simulink model "P2lab"  (Simulink 10.3)
settings: Solver=VariableStepAuto  StartTime=0.0  StopTime=Tfin  FixedStep=dt  MaxStep=dtmax  RelTol=1e-3  EnableMultiTasking=on
values from neighbouring files (symbols this model uses):
  a = 1    [P2_1b.m]    (also in P2_laboratorio.m)
  A0 = 1    [P2_1b.m]    (also in P2_laboratorio.m)
  b = 1    [P2_1b.m]    (also in P2_laboratorio.m = 0.666666666667)
  f0 = 1/20    (= 0.05)    [P2_1b.m]    (also in P2_laboratorio.m)
  T = 0.2    [P2_1b.m]    (also in P2_laboratorio.m = 0.737)
settings Model: Creator=anonimo  LastModifiedBy=34622  MultithreadedSim=on
settings SolverCC: ZeroCrossControl=EnableAll  AutoInsertRateTranBlk=on
settings DataIOCC: LimitDataPoints=on  SaveTime=off
settings DebuggingCC: SolverPrmCheckMsg=warning  SFExecutionAtInitializationDiag=warning

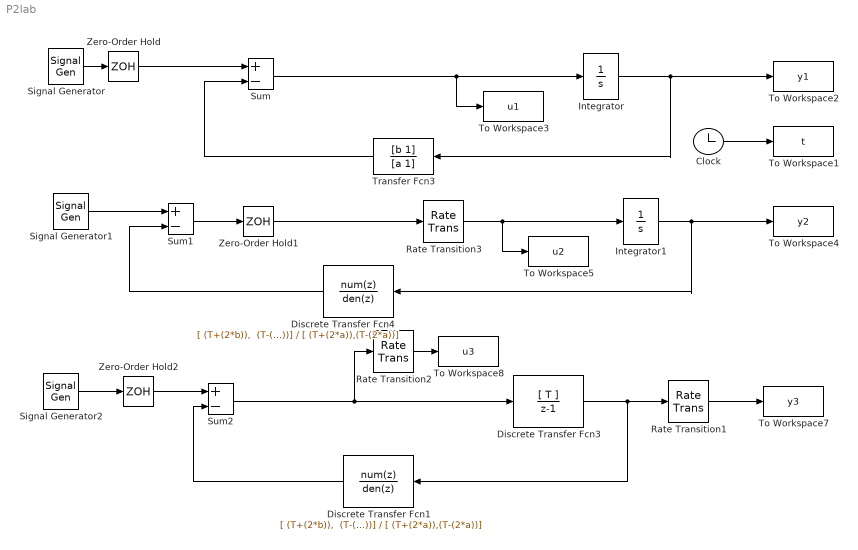
== system P2lab ==
  Clock : Clock
  Discrete Transfer Fcn1 : DiscreteTransferFcn  Numerator="[ (T+(2*b)),  (T-(2*b))]"  Denominator=[ (T+(2*a)),(T-(2*a))]  SampleTime=T
  Discrete Transfer Fcn3 : DiscreteTransferFcn  Numerator=[ T ]  Denominator="[ 1,  -1]"  SampleTime=T
  Discrete Transfer Fcn4 : DiscreteTransferFcn  Numerator="[ (T+(2*b)),  (T-(2*b))]"  Denominator=[ (T+(2*a)),(T-(2*a))]  SampleTime=T
  Integrator : Integrator
  Integrator1 : Integrator
  Rate Transition1 : RateTransition  Deterministic=off
  Rate Transition2 : RateTransition  Deterministic=off
  Rate Transition3 : RateTransition  Deterministic=off
  Signal Generator : SignalGenerator  WaveForm=square  Amplitude=A0  Frequency=f0
  Signal Generator1 : SignalGenerator  WaveForm=square  Amplitude=A0  Frequency=f0
  Signal Generator2 : SignalGenerator  WaveForm=square  Amplitude=A0  Frequency=f0
  Sum : Sum  Inputs=+-
  Sum1 : Sum  Inputs=+-
  Sum2 : Sum  Inputs=+-
  To Workspace1 : ToWorkspace  VariableName=t  SampleTime=-1
  To Workspace2 : ToWorkspace  VariableName=y1  SampleTime=-1
  To Workspace3 : ToWorkspace  VariableName=u1  SampleTime=-1
  To Workspace4 : ToWorkspace  VariableName=y2  SampleTime=-1
  To Workspace5 : ToWorkspace  VariableName=u2  SampleTime=-1
  To Workspace7 : ToWorkspace  VariableName=y3  SampleTime=-1
  To Workspace8 : ToWorkspace  VariableName=u3  SampleTime=-1
  Transfer Fcn3 : TransferFcn  Numerator=[b 1]  Denominator=[a 1]
  Zero-Order Hold : ZeroOrderHold  SampleTime=T
  Zero-Order Hold1 : ZeroOrderHold  SampleTime=T
  Zero-Order Hold2 : ZeroOrderHold  SampleTime=T
  wires:
  Integrator/1 -> Transfer Fcn3/1, To Workspace2/1
  Rate Transition3/1 -> To Workspace5/1, Integrator1/1
  Clock/1 -> To Workspace1/1
  Integrator1/1 -> Discrete Transfer Fcn4/1, To Workspace4/1
  Signal Generator/1 -> Zero-Order Hold/1
  Sum/1 -> Integrator/1, To Workspace3/1
  Zero-Order Hold1/1 -> Rate Transition3/1
  Sum1/1 -> Zero-Order Hold1/1
  Signal Generator1/1 -> Sum1/1
  Signal Generator2/1 -> Zero-Order Hold2/1
  Zero-Order Hold2/1 -> Sum2/1
  Sum2/1 -> Discrete Transfer Fcn3/1, Rate Transition2/1
  Discrete Transfer Fcn3/1 -> Discrete Transfer Fcn1/1, Rate Transition1/1
  Rate Transition1/1 -> To Workspace7/1
  Rate Transition2/1 -> To Workspace8/1
  Zero-Order Hold/1 -> Sum/1
  Transfer Fcn3/1 -> Sum/2
  Discrete Transfer Fcn4/1 -> Sum1/2
  Discrete Transfer Fcn1/1 -> Sum2/2
